simulink model "simpleControl"  (R2013a)
settings: Solver=FixedStepDiscrete  StartTime=0.0  StopTime=10.0  FixedStep=robot.Ts  RelTol=1e-3
values from neighbouring files (symbols this model uses):
  control = struct    [init.m]
  Reference = struct    [init.m]
undefined symbols (not defined in the file or in its folder): ROBOT_DOF
libraries: WBCLibrary x20, dspmtrx3 x2
settings Model: Creator=Raffaello  LastModifiedBy=Raffaello

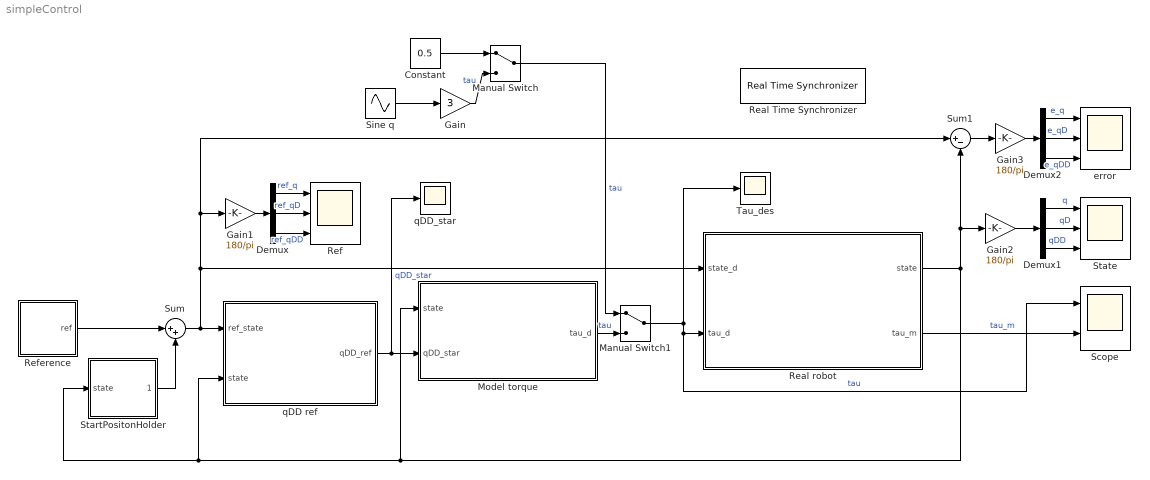
== system simpleControl ==
  Constant : Constant  Value=0.5
  Demux : Demux  Outputs=3
  Demux1 : Demux  Outputs=3
  Demux2 : Demux  Outputs=3
  Gain : Gain  Gain=3
  Gain1 : Gain  Gain=180/pi
  Gain2 : Gain  Gain=180/pi
  Gain3 : Gain  Gain=180/pi
  Manual Switch : ManualSwitch
  Manual Switch1 : ManualSwitch
  Model torque : Subsystem
  Real Time Synchronizer : WBCLibrary/Utilities/Real Time Synchronizer  Priority=-10  threadPeriod=Ts
  Real robot : Subsystem
  Ref : Scope  NumInputPorts=3
      settings: TimeRange=10  YMin=-80~-100~-300  YMax=-15~100~300
  Reference : Subsystem
  Scope : Scope  NumInputPorts=2
      settings: TimeRange=10  YMin=0.475~0.223  YMax=0.525~0.232
  Sine q : Sin  Amplitude=Reference.sinAmp  Bias=Reference.sinBias  Frequency=Reference.sinFreq*2*pi  SampleTime=0
  StartPositonHolder : Subsystem
  State : Scope  NumInputPorts=3
      settings: TimeRange=10  YMin=-65~-40~-400  YMax=-40~80~600  SaveName=ScopeData2
  Sum : Sum  Inputs=|++
  Sum1 : Sum  Inputs=|+-
  Tau_des : Scope
      settings: TimeRange=10  YMin=6  YMax=24  SaveName=ScopeData4
  error : Scope  NumInputPorts=3
      settings: TimeRange=10  YMin=-15~-80~-400  YMax=12.5~60~600  SaveName=ScopeData3
  qDD ref : Subsystem
  qDD_star : Scope
      settings: TimeRange=10  YMin=6  YMax=24  SaveName=ScopeData6
  wires:
  Manual Switch1/1 -> Scope/1, Real robot/2(tau_d), Tau_des/1  "tau"
  qDD ref/1(qDD_ref) -> qDD_star/1, Model torque/2(qDD_star)  "qDD_star"
  Real robot/2(tau_m) -> Scope/2  "tau_m"
  StartPositonHolder/1(state(0)) -> Sum/2
  Reference/1(ref) -> Sum/1
  Sum/1 -> Gain1/1, Sum1/1, Real robot/1(state_d), qDD ref/1(ref_state)
  Demux/2 -> Ref/2  "ref_qD"
  Demux/3 -> Ref/3  "ref_qDD"
  Real robot/1(state) -> StartPositonHolder/1(state), qDD ref/2(state), Model torque/1(state), Sum1/2, Gain2/1
  Demux1/1 -> State/1  "q"
  Demux1/2 -> State/2  "qD"
  Demux1/3 -> State/3  "qDD"
  Demux/1 -> Ref/1  "ref_q"
  Gain1/1 -> Demux/1
  Gain2/1 -> Demux1/1
  Demux2/2 -> error/2  "e_qD"
  Demux2/3 -> error/3  "e_qDD"
  Demux2/1 -> error/1  "e_q"
  Gain3/1 -> Demux2/1
  Sum1/1 -> Gain3/1
  Sine q/1 -> Gain/1
  Gain/1 -> Manual Switch/2  "tau"
  Constant/1 -> Manual Switch/1
  Model torque/1(tau_d) -> Manual Switch1/2  "tau"
  Manual Switch/1 -> Manual Switch1/1  "tau"

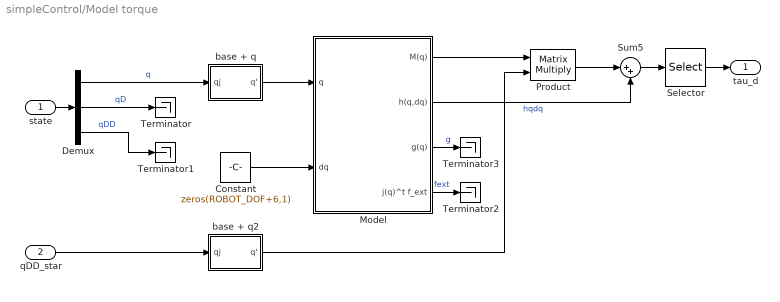
== system simpleControl/Model torque ==
  state : Inport
  qDD_star : Inport  Port=2
  Constant : Constant  Value=zeros(ROBOT_DOF+6,1)
  Demux : Demux  Outputs=3
  Model : Subsystem
  Product : Product  Multiplication=Matrix(*)
  Selector : Selector  InputPortWidth=ROBOT_DOF+6  IndexOptions=Index vector (dialog)  Indices=[7:ROBOT_DOF+6]  OutputSizes=1
  Sum5 : Sum  Inputs=|++
  Terminator{,1..3} (4 alike) : Terminator
  base + q : Subsystem
  base + q2 : Subsystem
  tau_d : Outport
  wires:
  Product/1 -> Sum5/1
  Model/2(h(q,dq)) -> Sum5/2  "hqdq"
  qDD_star/1 -> base + q2/1(qj)
  Model/4(j(q)^t f_ext) -> Terminator2/1  "fext"
  base + q/1(q') -> Model/1(q)
  Model/3(g(q)) -> Terminator3/1  "g"
  Model/1(M(q)) -> Product/1
  Constant/1 -> Model/2(dq)
  Sum5/1 -> Selector/1
  base + q2/1(q') -> Product/2
  state/1 -> Demux/1
  Demux/1 -> base + q/1(qj)  "q"
  Demux/2 -> Terminator/1  "qD"
  Demux/3 -> Terminator1/1  "qDD"
  Selector/1 -> tau_d/1

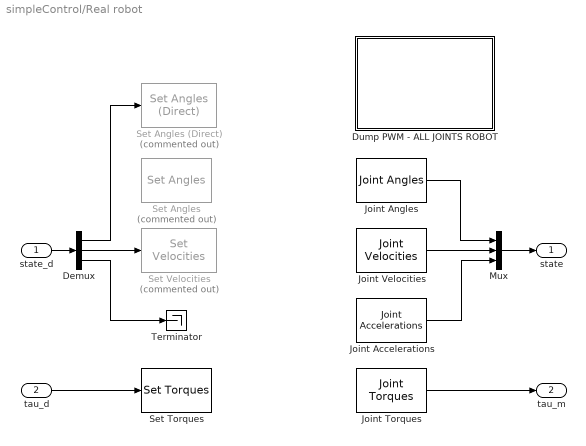
== system simpleControl/Real robot ==
  state_d : Inport
  tau_d : Inport  Port=2
  Demux : Demux  Outputs=3
  Dump PWM - ALL JOINTS ROBOT : Subsystem  mask{output='getOutputs'}
      mask prompts: output "Output port"
      mask Display:
      | color('red'); plot([10 20 30 40], [10 20 10 15]);
      | color('blue'); plot([10 20 30 40], [15 10 20 12]);
      | color('green'); plot([10 20 30 40], [13 16 12 18]);
  Joint Accelerations : WBCLibrary/wholeBodyStates/Joint Accelerations  robotName=robot.robotName  localName=robot.localName
  Joint Angles : WBCLibrary/wholeBodyStates/Joint Angles  robotName=robot.robotName  localName=robot.localName
  Joint Torques : WBCLibrary/wholeBodyStates/Joint Torques  robotName=robot.robotName  localName=robot.localName
  Joint Velocities : WBCLibrary/wholeBodyStates/Joint Velocities  robotName=robot.robotName  localName=robot.localName
  Mux : Mux  Inputs=3
  Set Angles : WBCLibrary/wholeBodyActuators/Set Angles  Commented=on  val=5  robotName=robot.robotName  localName=robot.localName
  Set Angles (Direct) : WBCLibrary/wholeBodyActuators/Set Angles (Direct)  Commented=on  val=20  robotName=robot.robotName  localName=robot.localName
  Set Torques : WBCLibrary/wholeBodyActuators/Set Torques  val=6  robotName=robot.robotName  localName=robot.localName
  Set Velocities : WBCLibrary/wholeBodyActuators/Set Velocities  Commented=on  val=4  robotName=robotName  localName=localName
  Terminator : Terminator
  state : Outport
  tau_m : Outport  Port=2
  wires:
  Joint Velocities/1 -> Mux/2
  tau_d/1 -> Set Torques/1
  Joint Accelerations/1 -> Mux/3
  Joint Angles/1 -> Mux/1
  Mux/1 -> state/1
  Joint Torques/1 -> tau_m/1
  state_d/1 -> Demux/1
  Demux/1 -> Set Angles (Direct)/1
  Demux/2 -> Set Velocities/1
  Demux/3 -> Terminator/1

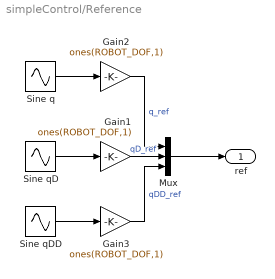
== system simpleControl/Reference ==
  Gain1 : Gain  Gain=ones(ROBOT_DOF,1)
  Gain2 : Gain  Gain=ones(ROBOT_DOF,1)
  Gain3 : Gain  Gain=ones(ROBOT_DOF,1)
  Mux : Mux  Inputs=3
  Sine q : Sin  Amplitude=Reference.sinAmp  Bias=Reference.sinBias  Frequency=Reference.sinFreq*2*pi  SampleTime=0
  Sine qD : Sin  Amplitude=Reference.sinAmp*Reference.sinFreq*2*pi  Frequency=Reference.sinFreq*2*pi  Phase=pi/2  SampleTime=0
  Sine qDD : Sin  Amplitude=-Reference.sinAmp*(Reference.sinFreq*2*pi)^2  Frequency=Reference.sinFreq*2*pi  SampleTime=0
  ref : Outport
  wires:
  Sine q/1 -> Gain2/1
  Sine qD/1 -> Gain1/1
  Sine qDD/1 -> Gain3/1
  Mux/1 -> ref/1
  Gain2/1 -> Mux/1  "q_ref"
  Gain1/1 -> Mux/2  "qD_ref"
  Gain3/1 -> Mux/3  "qDD_ref"

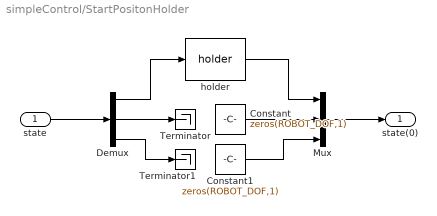
== system simpleControl/StartPositonHolder ==
  state : Inport
  Constant : Constant  Value=zeros(ROBOT_DOF,1)
  Constant1 : Constant  Value=zeros(ROBOT_DOF,1)
  Demux : Demux  Outputs=3
  Mux : Mux  Inputs=3
  Terminator : Terminator
  Terminator1 : Terminator
  "holder " : WBCLibrary/Utilities/holder 
  state(0) : Outport
  wires:
  Demux/1 -> "holder "/1
  state/1 -> Demux/1
  Mux/1 -> state(0)/1
  "holder "/1 -> Mux/1
  Demux/2 -> Terminator/1
  Demux/3 -> Terminator1/1
  Constant/1 -> Mux/2
  Constant1/1 -> Mux/3

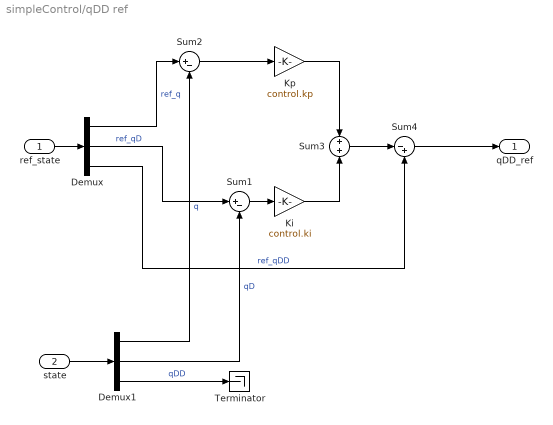
== system simpleControl/qDD ref ==
  ref_state : Inport
  state : Inport  Port=2
  Demux : Demux  Outputs=3
  Demux1 : Demux  Outputs=3
  Ki : Gain  Gain=control.ki
  Kp : Gain  Gain=control.kp
  Sum1 : Sum  Inputs=|+-
  Sum2 : Sum  Inputs=|+-
  Sum3 : Sum
  Sum4 : Sum  Inputs=|-+
  Terminator : Terminator
  qDD_ref : Outport
  wires:
  Demux/1 -> Sum2/1  "ref_q"
  Kp/1 -> Sum3/1
  Sum3/1 -> Sum4/1
  Demux1/1 -> Sum2/2  "q"
  Sum2/1 -> Kp/1
  Sum4/1 -> qDD_ref/1
  Sum1/1 -> Ki/1
  Demux1/2 -> Sum1/2  "qD"
  Demux/3 -> Sum4/2  "ref_qDD"
  ref_state/1 -> Demux/1
  state/1 -> Demux1/1
  Demux1/3 -> Terminator/1  "qDD"
  Ki/1 -> Sum3/2
  Demux/2 -> Sum1/1  "ref_qD"

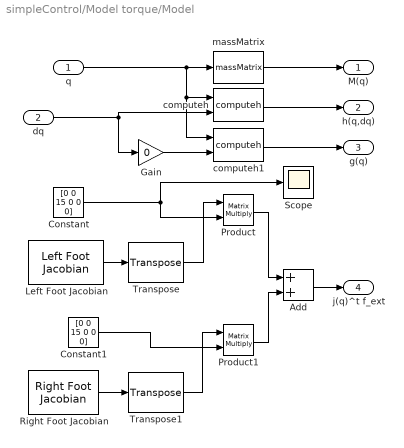
== system simpleControl/Model torque/Model ==
  q : Inport
  dq : Inport  Port=2
  Add : Sum
  Constant : Constant  Value=[0 0 15 0 0 0]
  Constant1 : Constant  Value=[0 0 15 0 0 0]
  Gain : Gain  Gain=0
  Left Foot Jacobian : WBCLibrary/wholeBodyModel/Jacobians/Left Foot Jacobian  robotName=robot.robotName  localName=robot.localName
  Product : Product  Multiplication=Matrix(*)
  Product1 : Product  Multiplication=Matrix(*)
  Right Foot Jacobian : WBCLibrary/wholeBodyModel/Jacobians/Right Foot Jacobian  robotName=robot.robotName  localName=robot.localName
  Scope : Scope
  Transpose : dspmtrx3/Transpose  Hermitian=off  overflowFlag=off
  Transpose1 : dspmtrx3/Transpose  Hermitian=off  overflowFlag=off
  computeh : WBCLibrary/wholeBodyModel/Dynamics/computeh  val=7  robotname=robot.robotName  localname=robot.localName
  computeh1 : WBCLibrary/wholeBodyModel/Dynamics/computeh  val=7  robotname=robot.robotName  localname=robot.localName
  massMatrix : WBCLibrary/wholeBodyModel/Dynamics/massMatrix  val=8  robotname=robot.robotName  localname=robot.localName
  M(q) : Outport
  h(q,dq) : Outport  Port=2
  g(q) : Outport  Port=3
  j(q)^t f_ext : Outport  Port=4
  wires:
  Gain/1 -> computeh1/2
  computeh1/1 -> g(q)/1
  computeh/1 -> h(q,dq)/1
  massMatrix/1 -> M(q)/1
  q/1 -> computeh1/1, computeh/1, massMatrix/1
  dq/1 -> computeh/2, Gain/1
  Left Foot Jacobian/1 -> Transpose/1
  Right Foot Jacobian/1 -> Transpose1/1
  Constant/1 -> Product/2, Scope/1
  Transpose/1 -> Product/1
  Constant1/1 -> Product1/2
  Transpose1/1 -> Product1/1
  Product/1 -> Add/1
  Product1/1 -> Add/2
  Add/1 -> j(q)^t f_ext/1

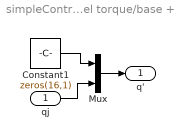
== system simpleControl/Model torque/base + q ==
  qj : Inport
  Constant1 : Constant  Value=zeros(16,1)
  Mux : Mux  Inputs=2
  q' : Outport
  wires:
  Mux/1 -> q'/1
  qj/1 -> Mux/2
  Constant1/1 -> Mux/1

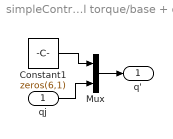
== system simpleControl/Model torque/base + q2 ==
  qj : Inport
  Constant1 : Constant  Value=zeros(6,1)
  Mux : Mux  Inputs=2
  q' : Outport
  wires:
  Constant1/1 -> Mux/1
  qj/1 -> Mux/2
  Mux/1 -> q'/1

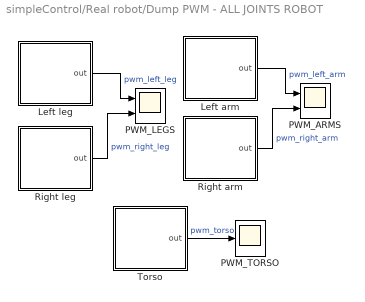
== system simpleControl/Real robot/Dump PWM - ALL JOINTS ROBOT ==
  Left arm : Subsystem  mask{type_arm='left_arm', output=output}
      mask prompts: type_arm "Type leg"; output "Output Port"
  Left leg : Subsystem  mask{type_arm='left_leg', output=output}
      mask prompts: type_arm "Type leg"; output "Output port"
  PWM_ARMS : Scope  NumInputPorts=2
      settings: TimeRange=60  YMin=-10~-10  YMax=12.5~15
  PWM_LEGS : Scope  NumInputPorts=2
      settings: TimeRange=10  YMin=-1~-7.5  YMax=1~22.5
  PWM_TORSO : Scope
      settings: TimeRange=60  YMin=-10  YMax=12.5  SaveName=ScopeData5
  Right arm : Subsystem  mask{type_arm='right_arm', output=output}
      mask prompts: type_arm "Type leg"; output "Output Port"
  Right leg : Subsystem  mask{type_arm='right_leg', output=output}
      mask prompts: type_arm "Type leg"; output "Output port"
  Torso : Subsystem  mask{type_arm='torso', output=output}
      mask prompts: type_arm "Type leg"; output "Output port"
  wires:
  Left arm/1(out) -> PWM_ARMS/1  "pwm_left_arm"
  Right arm/1(out) -> PWM_ARMS/2  "pwm_right_arm"
  Torso/1(out) -> PWM_TORSO/1  "pwm_torso"
  Right leg/1(out) -> PWM_LEGS/2  "pwm_right_leg"
  Left leg/1(out) -> PWM_LEGS/1  "pwm_left_leg"

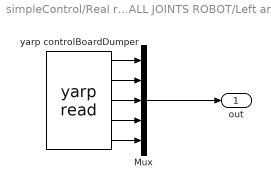
== system simpleControl/Real robot/Dump PWM - ALL JOINTS ROBOT/Left arm ==
  Mux : Mux  Inputs=5
  yarp controlBoardDumper : WBCLibrary/Utilities/yarp read  from=['/controlBoardDumper/' type_arm '/' output]  to='...'  num=5  blocking=off  timestamp=off
  out : Outport
  wires:
  Mux/1 -> out/1
  yarp controlBoardDumper/1 -> Mux/1
  yarp controlBoardDumper/3 -> Mux/3
  yarp controlBoardDumper/2 -> Mux/2
  yarp controlBoardDumper/5 -> Mux/5
  yarp controlBoardDumper/4 -> Mux/4

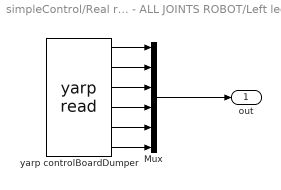
== system simpleControl/Real robot/Dump PWM - ALL JOINTS ROBOT/Left leg ==
  Mux : Mux  Inputs=6
  yarp controlBoardDumper : WBCLibrary/Utilities/yarp read  from=['/controlBoardDumper/' type_arm '/' output]  to='...'  num=6  blocking=off  timestamp=off
  out : Outport
  wires:
  Mux/1 -> out/1
  yarp controlBoardDumper/1 -> Mux/1
  yarp controlBoardDumper/3 -> Mux/3
  yarp controlBoardDumper/2 -> Mux/2
  yarp controlBoardDumper/5 -> Mux/5
  yarp controlBoardDumper/6 -> Mux/6
  yarp controlBoardDumper/4 -> Mux/4

== system simpleControl/Real robot/Dump PWM - ALL JOINTS ROBOT/Right arm ==
  Mux : Mux  Inputs=5
  yarp controlBoardDumper : WBCLibrary/Utilities/yarp read  from=['/controlBoardDumper/' type_arm '/' output]  to='...'  num=5  blocking=off  timestamp=off
  out : Outport
  wires:
  Mux/1 -> out/1
  yarp controlBoardDumper/1 -> Mux/1
  yarp controlBoardDumper/3 -> Mux/3
  yarp controlBoardDumper/2 -> Mux/2
  yarp controlBoardDumper/5 -> Mux/5
  yarp controlBoardDumper/4 -> Mux/4

== system simpleControl/Real robot/Dump PWM - ALL JOINTS ROBOT/Right leg ==
  Mux : Mux  Inputs=6
  yarp controlBoardDumper : WBCLibrary/Utilities/yarp read  from=['/controlBoardDumper/' type_arm '/' output]  to='...'  num=6  blocking=off  timestamp=off
  out : Outport
  wires:
  Mux/1 -> out/1
  yarp controlBoardDumper/1 -> Mux/1
  yarp controlBoardDumper/3 -> Mux/3
  yarp controlBoardDumper/2 -> Mux/2
  yarp controlBoardDumper/5 -> Mux/5
  yarp controlBoardDumper/6 -> Mux/6
  yarp controlBoardDumper/4 -> Mux/4

== system simpleControl/Real robot/Dump PWM - ALL JOINTS ROBOT/Torso ==
  Mux : Mux  Inputs=3
  yarp controlBoardDumper : WBCLibrary/Utilities/yarp read  from=['/controlBoardDumper/' type_arm '/' output]  to='...'  num=3  blocking=off  timestamp=off
  out : Outport
  wires:
  Mux/1 -> out/1
  yarp controlBoardDumper/1 -> Mux/1
  yarp controlBoardDumper/3 -> Mux/3
  yarp controlBoardDumper/2 -> Mux/2
